simulink model "homework2Simulink"  (R2018b)
settings: Solver=VariableStepAuto  StartTime=0.0  StopTime=tsim  MaxStep=1e-4  RelTol=1e-4
undefined symbols (not defined in the file or in its folder): dist1, dist2, kc1, kc2, kr1, kr2, ref11, ref12, ref21, ref22, tref11, tref12, tref21, tref22, Ts
libraries: cstblocks x2
settings Model: Creator=fvani  LastModifiedBy=fvani

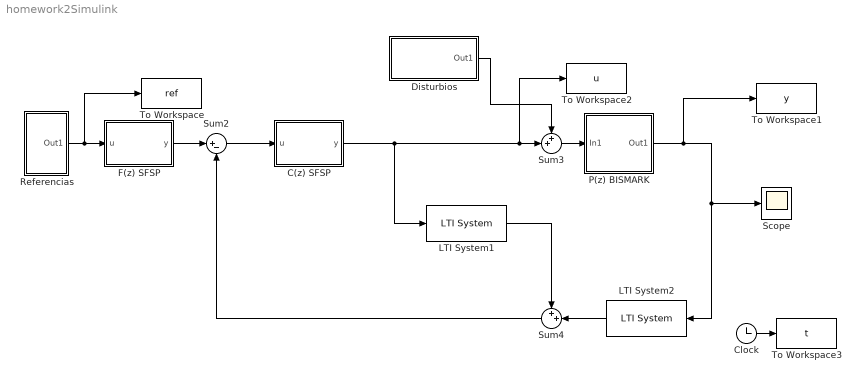
== system homework2Simulink ==
  C(z) SFSP : Subsystem
  Clock : Clock
  Disturbios : Subsystem
  F(z) SFSP : Subsystem
  LTI System1 : cstblocks/LTI System  sys=S  IC=[]
  LTI System2 : cstblocks/LTI System  sys=V  IC=[]
  P(z) BISMARK : Subsystem
  Referencias : Subsystem
  Scope : Scope
  Sum2 : Sum  Inputs=|+-
  Sum3 : Sum  Inputs=++|
  Sum4 : Sum  Inputs=++|
  To Workspace : ToWorkspace  VariableName=ref  SampleTime=-1
  To Workspace1 : ToWorkspace  VariableName=y  SampleTime=-1
  To Workspace2 : ToWorkspace  VariableName=u  SampleTime=-1
  To Workspace3 : ToWorkspace  VariableName=t  SampleTime=Ts
  wires:
  F(z) SFSP/1(y) -> Sum2/1
  Sum2/1 -> C(z) SFSP/1(u)
  Sum3/1 -> P(z) BISMARK/1(In1)
  P(z) BISMARK/1(Out1) -> LTI System2/1, Scope/1, To Workspace1/1
  LTI System2/1 -> Sum4/2
  Sum4/1 -> Sum2/2
  Referencias/1(Out1) -> To Workspace/1, F(z) SFSP/1(u)
  Disturbios/1(Out1) -> Sum3/1
  Clock/1 -> To Workspace3/1
  C(z) SFSP/1(y) -> LTI System1/1, To Workspace2/1, Sum3/2
  LTI System1/1 -> Sum4/1

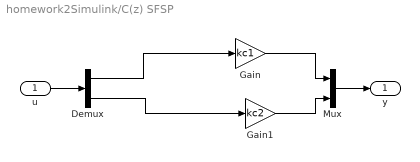
== system homework2Simulink/C(z) SFSP ==
  u : Inport
  Demux : Demux  Outputs=2
  Gain : Gain  Gain=kc1
  Gain1 : Gain  Gain=kc2
  Mux : Mux  Inputs=2
  y : Outport
  wires:
  Demux/1 -> Gain/1
  Gain/1 -> Mux/1
  u/1 -> Demux/1
  Mux/1 -> y/1
  Demux/2 -> Gain1/1
  Gain1/1 -> Mux/2

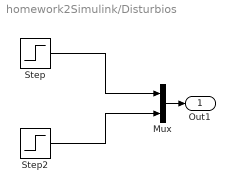
== system homework2Simulink/Disturbios ==
  Mux : Mux  Inputs=2
  Step : Step  Time=dist1  After=-0.1  SampleTime=Ts
  Step2 : Step  Time=dist2  After=0.1  SampleTime=Ts
  Out1 : Outport
  wires:
  Mux/1 -> Out1/1
  Step2/1 -> Mux/2
  Step/1 -> Mux/1

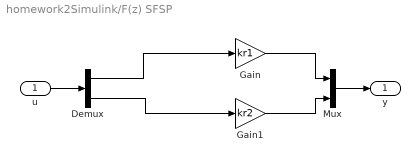
== system homework2Simulink/F(z) SFSP ==
  u : Inport
  Demux : Demux  Outputs=2
  Gain : Gain  Gain=kr1
  Gain1 : Gain  Gain=kr2
  Mux : Mux  Inputs=2
  y : Outport
  wires:
  Demux/1 -> Gain/1
  Gain/1 -> Mux/1
  u/1 -> Demux/1
  Mux/1 -> y/1
  Demux/2 -> Gain1/1
  Gain1/1 -> Mux/2

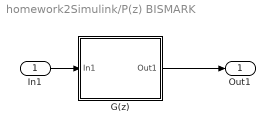
== system homework2Simulink/P(z) BISMARK ==
  In1 : Inport
  G(z) : Subsystem
  Out1 : Outport
  wires:
  In1/1 -> G(z)/1(In1)
  G(z)/1(Out1) -> Out1/1

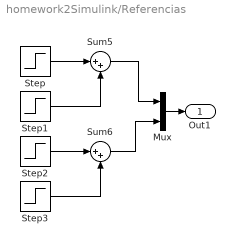
== system homework2Simulink/Referencias ==
  Mux : Mux  Inputs=2
  Step : Step  Time=tref11  After=ref11  SampleTime=Ts
  Step1 : Step  Time=tref12  After=ref12  SampleTime=Ts
  Step2 : Step  Time=tref21  After=ref21  SampleTime=Ts
  Step3 : Step  Time=tref22  After=ref22  SampleTime=Ts
  Sum5 : Sum  Inputs=|++
  Sum6 : Sum  Inputs=|++
  Out1 : Outport
  wires:
  Step/1 -> Sum5/1
  Step2/1 -> Sum6/1
  Step1/1 -> Sum5/2
  Step3/1 -> Sum6/2
  Sum5/1 -> Mux/1
  Sum6/1 -> Mux/2
  Mux/1 -> Out1/1

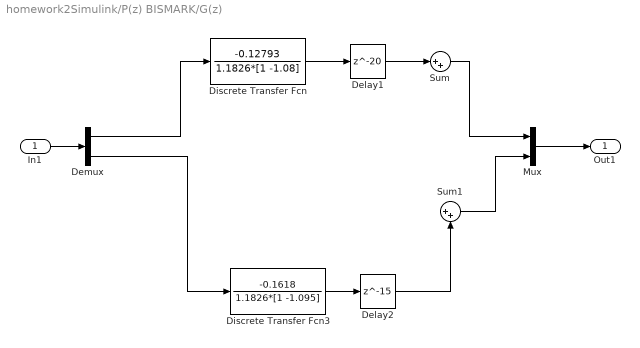
== system homework2Simulink/P(z) BISMARK/G(z) ==
  In1 : Inport
  Delay1 : Delay  DelayLength=20  SampleTime=Ts
  Delay2 : Delay  DelayLength=15  SampleTime=Ts
  Demux : Demux  Outputs=2
  Discrete Transfer Fcn : DiscreteTransferFcn  Numerator=-0.12793  Denominator=1.1826*[1 -1.08]  SampleTime=Ts
  Discrete Transfer Fcn3 : DiscreteTransferFcn  Numerator=-0.1618  Denominator=1.1826*[1 -1.095]  SampleTime=Ts
  Mux : Mux  Inputs=2
  Sum : Sum  Inputs=|++
  Sum1 : Sum  Inputs=|++
  Out1 : Outport
  wires:
  Demux/1 -> Discrete Transfer Fcn/1
  In1/1 -> Demux/1
  Demux/2 -> Discrete Transfer Fcn3/1
  Sum/1 -> Mux/1
  Discrete Transfer Fcn/1 -> Delay1/1
  Discrete Transfer Fcn3/1 -> Delay2/1
  Sum1/1 -> Mux/2
  Mux/1 -> Out1/1
  Delay1/1 -> Sum/1
  Delay2/1 -> Sum1/2
